simulink model "Roll_Autopilot_PP"  (R2017b)
settings: Solver=FixedStepDiscrete  StartTime=0.0  StopTime=10.0  FixedStep=0.025000  RelTol=1e-3
model workspace (MAT data in the model file):
  MCOS : class17 (value not decoded)
  already_pp = 1
  compositionalMap : struct (value not decoded)
  MCOS : class17 (value not decoded)
  MCOS : class17 (value not decoded)
  verificationResults : struct (value not decoded)
undefined symbols (not defined in the file): contractAfterSimulation, contractBeforeSimulation, ContractBlock, ContractEnsureBlock, ContractGuaranteeBlock, ContractModeBlock, ContractRequireBlock, ContractValidatorBlock, pp_lib, saturation, saveValidatorParameters, slcm, Ts
(part 2 of 3)

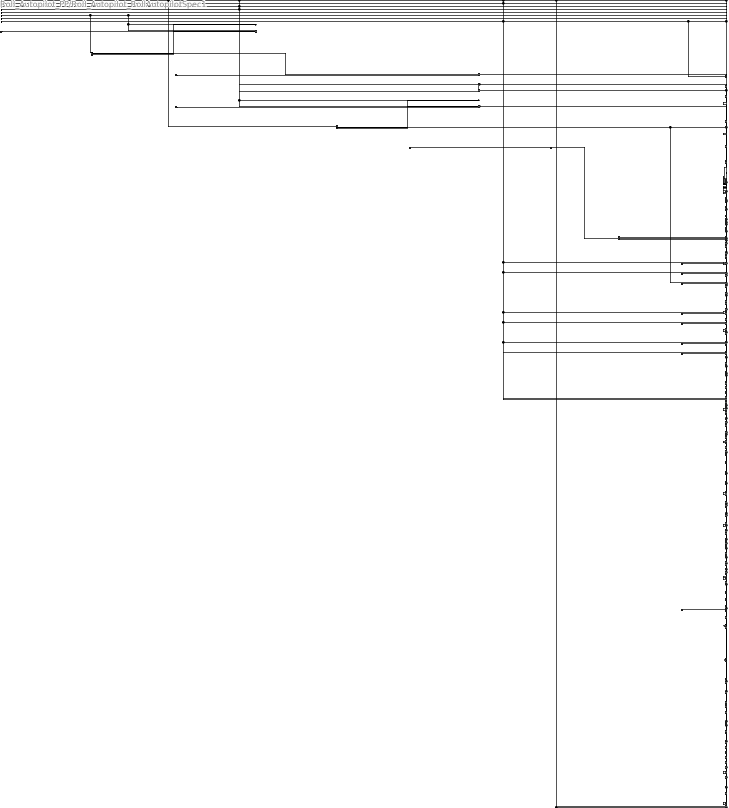
== system Roll_Autopilot_PP/Roll_Autopilot_RollAutopilotSpec1 ==
  note: contract has non-exhaustive modes
  RollAutopilotSpec_roll_angle : Inport  OutDataTypeStr=double
  RollAutopilotSpec_TurnKnob : Inport  Port=2  OutDataTypeStr=double
  RollAutopilotSpec_HDGmode : Inport  Port=3  OutDataTypeStr=boolean
  RollAutopilotSpec_autopilot_engaged : Inport  Port=4  OutDataTypeStr=boolean
  RollAutopilotSpec_hdg_hold_mode_cmd : Inport  Port=5  OutDataTypeStr=double
  RollAutopilotSpec_roll_actuator_command : Inport  Port=6  OutDataTypeStr=double
  RollAutopilotSpec_roll_cmd : Inport  Port=7  OutDataTypeStr=double
  RollAutopilotSpec_roll_hold_reference : Inport  Port=8  OutDataTypeStr=double
  AP_minus_001 : Subsystem  TreatAsAtomicUnit=on  mask(ContractGuaranteeBlock){ContractBlockType=ContractGuaranteeBlock}
      mask init:
      | set_param(gcb, 'LinkStatus', 'none');
      mask DialogControl DescTextVar Prompt: Guarantee block
  AP_minus_003A : Subsystem  TreatAsAtomicUnit=on  mask(ContractGuaranteeBlock){ContractBlockType=ContractGuaranteeBlock}
      mask init:
      | set_param(gcb, 'LinkStatus', 'none');
      mask DialogControl DescTextVar Prompt: Guarantee block
      mask DialogControl Display_counter_example_as_signals Prompt: Display counter example as signals
      mask DialogControl Display_counter_example_as_signals Callback: displayCexSignals(3, 4);displayCexSignals(2,
      mask DialogControl Display_counter_example_as_tables Prompt: Display counter example as tables
      mask DialogControl Display_counter_example_as_tables Callback: displayCexTables(3, 4);displayCexTables(2,
      mask DialogControl Display_counter_example_as_HTML_tables Prompt: Display counter example as HTML tables
      mask DialogControl Display_counter_example_as_HTML_tables Callback: displayCexHtmlTables(3, 4);displayCexHtmlTables(2,
      mask DialogControl Generate_an_outer_model_for_the_counter_example Prompt: Generate an outer model for the counter example
      mask DialogControl Generate_an_outer_model_for_the_counter_example Callback: generateModelWithSignalBuilders(3, 4, 2);generateModelWithSignalBuilders(2,
      mask DialogControl Generate_an_inner_model_for_the_counter_example Prompt: Generate an inner model for the counter example
      mask DialogControl Generate_an_inner_model_for_the_counter_example Callback: generateModelWithSignalBuilders(3, 4, 1);generateModelWithSignalBuilders(2,
  AP_minus_003B : Subsystem  TreatAsAtomicUnit=on  mask(ContractGuaranteeBlock){ContractBlockType=ContractGuaranteeBlock}
      mask init:
      | set_param(gcb, 'LinkStatus', 'none');
      mask DialogControl DescTextVar Prompt: Guarantee block
      mask DialogControl Display_counter_example_as_signals Prompt: Display counter example as signals
      mask DialogControl Display_counter_example_as_signals Callback: displayCexSignals(3, 4);displayCexSignals(1,
      mask DialogControl Display_counter_example_as_tables Prompt: Display counter example as tables
      mask DialogControl Display_counter_example_as_tables Callback: displayCexTables(3, 4);displayCexTables(1,
      mask DialogControl Display_counter_example_as_HTML_tables Prompt: Display counter example as HTML tables
      mask DialogControl Display_counter_example_as_HTML_tables Callback: displayCexHtmlTables(3, 4);displayCexHtmlTables(1,
      mask DialogControl Generate_an_outer_model_for_the_counter_example Prompt: Generate an outer model for the counter example
      mask DialogControl Generate_an_outer_model_for_the_counter_example Callback: generateModelWithSignalBuilders(3, 4, 2);generateModelWithSignalBuilders(1,
      mask DialogControl Generate_an_inner_model_for_the_counter_example Prompt: Generate an inner model for the counter example
      mask DialogControl Generate_an_inner_model_for_the_counter_example Callback: generateModelWithSignalBuilders(3, 4, 1);generateModelWithSignalBuilders(1,
  AP_minus_003C : Subsystem  TreatAsAtomicUnit=on  mask(ContractGuaranteeBlock){ContractBlockType=ContractGuaranteeBlock}
      mask init:
      | set_param(gcb, 'LinkStatus', 'none');
      mask DialogControl DescTextVar Prompt: Guarantee block
      mask DialogControl Display_counter_example_as_signals Prompt: Display counter example as signals
      mask DialogControl Display_counter_example_as_signals Callback: displayCexSignals(3, 4);displayCexSignals(3,
      mask DialogControl Display_counter_example_as_tables Prompt: Display counter example as tables
      mask DialogControl Display_counter_example_as_tables Callback: displayCexTables(3, 4);displayCexTables(3,
      mask DialogControl Display_counter_example_as_HTML_tables Prompt: Display counter example as HTML tables
      mask DialogControl Display_counter_example_as_HTML_tables Callback: displayCexHtmlTables(3, 4);displayCexHtmlTables(3,
      mask DialogControl Generate_an_outer_model_for_the_counter_example Prompt: Generate an outer model for the counter example
      mask DialogControl Generate_an_outer_model_for_the_counter_example Callback: generateModelWithSignalBuilders(3, 4, 2);generateModelWithSignalBuilders(3,
      mask DialogControl Generate_an_inner_model_for_the_counter_example Prompt: Generate an inner model for the counter example
      mask DialogControl Generate_an_inner_model_for_the_counter_example Callback: generateModelWithSignalBuilders(3, 4, 1);generateModelWithSignalBuilders(3,
  AP_minus_003D : Subsystem  TreatAsAtomicUnit=on  mask(ContractGuaranteeBlock){ContractBlockType=ContractGuaranteeBlock}
      mask init:
      | set_param(gcb, 'LinkStatus', 'none');
      mask DialogControl DescTextVar Prompt: Guarantee block
  AP_minus_007 : Subsystem  TreatAsAtomicUnit=on  mask(ContractGuaranteeBlock){ContractBlockType=ContractGuaranteeBlock}
      mask init:
      | set_param(gcb, 'LinkStatus', 'none');
      mask DialogControl DescTextVar Prompt: Guarantee block
  Arrow_xxRollAutopilotSpec_162_ni_7 : Delay  DelayLength=1  InitialCondition=1
  Arrow_xxRollAutopilotSpec_163_ni_9 : Delay  DelayLength=1  InitialCondition=1
  Arrow_xxRollAutopilotSpec_164_ni_12 : Delay  DelayLength=1  InitialCondition=1
  Arrow_xxRollAutopilotSpec_165_ni_16 : Delay  DelayLength=1  InitialCondition=1
  Arrow_xxRollAutopilotSpec_183_ni_3 : Delay  DelayLength=1  InitialCondition=1
  Ca_operator : Logic  Operator=NOT  AllPortsSameDT=off  OutDataTypeStr=boolean
  Cb_operator : Logic  AllPortsSameDT=off  OutDataTypeStr=boolean
  Cc_operator : RelationalOperator  OutDataTypeStr=boolean  RndMeth=Simplest
  Cc_rhs_2 : Constant  Value=30.0  OutDataTypeStr=double
  Cd_operator : Logic  AllPortsSameDT=off  OutDataTypeStr=boolean
  H_call : Subsystem  TreatAsAtomicUnit=on
  H_call1 : Subsystem  TreatAsAtomicUnit=on
  H_call11 : Subsystem  TreatAsAtomicUnit=on
  PRE_xxRollAutopilotSpec_{8,13,17,22,33,38,42,44,59,64,68,73,84,89,93,95,109,114,118,123,133,138,142,144,184,187} (26 alike) : Delay  DelayLength=1  InitialCondition=0
  SI_call : Subsystem  TreatAsAtomicUnit=on
  SI_call1 : Subsystem  TreatAsAtomicUnit=on
  SI_call11 : Subsystem  TreatAsAtomicUnit=on
  SI_call111 : Subsystem  TreatAsAtomicUnit=on
  SI_call1111 : Subsystem  TreatAsAtomicUnit=on
  SI_call11111 : Subsystem  TreatAsAtomicUnit=on
  SI_call111111 : Subsystem  TreatAsAtomicUnit=on
  SI_call1111111 : Subsystem  TreatAsAtomicUnit=on
  SI_call11111111 : Subsystem  TreatAsAtomicUnit=on
  branch_10_IF : Switch  Criteria=u2 ~= 0
  branch_11_IF : Switch  Criteria=u2 ~= 0
  branch_12_IF : Switch  Criteria=u2 ~= 0
  branch_13_IF : Switch  Criteria=u2 ~= 0
  branch_14_IF : Switch  Criteria=u2 ~= 0
  branch_15_IF : Switch  Criteria=u2 ~= 0
  branch_16_IF : Switch  Criteria=u2 ~= 0
  branch_8_IF : Switch  Criteria=u2 ~= 0
  branch_9_IF : Switch  Criteria=u2 ~= 0
  hdg_hold_mode : Subsystem  TreatAsAtomicUnit=on  mask(ContractModeBlock){ContractBlockType=ContractModeBlock}
      mask init:
      | set_param(gcb, 'LinkStatus', 'none');
      mask DialogControl DescTextVar Prompt: Mode block
  hdg_hold_mode_ensure : Subsystem  TreatAsAtomicUnit=on  mask(ContractEnsureBlock){ContractBlockType=ContractEnsureBlock}
      mask init:
      | set_param(gcb, 'LinkStatus', 'none');
      mask DialogControl DescTextVar Prompt: Ensure block
  hdg_hold_mode_ensure_cond : Logic  Inputs=1  AllPortsSameDT=off  OutDataTypeStr=boolean
  hdg_hold_mode_require : Subsystem  TreatAsAtomicUnit=on  mask(ContractRequireBlock){ContractBlockType=ContractRequireBlock}
      mask init:
      | set_param(gcb, 'LinkStatus', 'none');
      mask DialogControl DescTextVar Prompt: Require block
  hdg_hold_mode_require_cond : Logic  Inputs=1  AllPortsSameDT=off  OutDataTypeStr=boolean
  no_other_lateral_mode_operator : Logic  Operator=NOT  AllPortsSameDT=off  OutDataTypeStr=boolean
  roll_hold_mode : Subsystem  TreatAsAtomicUnit=on  mask(ContractModeBlock){ContractBlockType=ContractModeBlock}
      mask init:
      | set_param(gcb, 'LinkStatus', 'none');
      mask DialogControl DescTextVar Prompt: Mode block
  roll_hold_mode_ensure : Subsystem  TreatAsAtomicUnit=on  mask(ContractEnsureBlock){ContractBlockType=ContractEnsureBlock}
      mask init:
      | set_param(gcb, 'LinkStatus', 'none');
      mask DialogControl DescTextVar Prompt: Ensure block
  roll_hold_mode_ensure_cond : Logic  Inputs=1  AllPortsSameDT=off  OutDataTypeStr=boolean
  roll_hold_mode_require : Subsystem  TreatAsAtomicUnit=on  mask(ContractRequireBlock){ContractBlockType=ContractRequireBlock}
      mask init:
      | set_param(gcb, 'LinkStatus', 'none');
      mask DialogControl DescTextVar Prompt: Require block
  roll_hold_mode_require_cond : Logic  Inputs=1  AllPortsSameDT=off  OutDataTypeStr=boolean
  roll_hold_operator : Logic  AllPortsSameDT=off  OutDataTypeStr=boolean
  spec206_operator : Subsystem  TreatAsAtomicUnit=on
  spec211_operator : Logic  AllPortsSameDT=off  OutDataTypeStr=boolean
  spec216_operator : RelationalOperator  Operator===  OutDataTypeStr=boolean  RndMeth=Simplest
  spec223_operator : RelationalOperator  Operator===  OutDataTypeStr=boolean  RndMeth=Simplest
  spec252_operator : Subsystem  TreatAsAtomicUnit=on
  spec621_operator : RelationalOperator  Operator=<=  OutDataTypeStr=boolean  RndMeth=Simplest
  spec621_rhs_2 : Constant  Value=15.0  OutDataTypeStr=double
  validator : M-S-Function  LoadFcn=saveValidatorParameters(gcb);  InitFcn=contractBeforeSimulation();  StopFcn=contractAfterSimulation();  FunctionName=contract  mask(ContractValidatorBlock){assumePorts=0, guaranteePorts=6, modePorts=2, ContractBlockType=ContractValidatorBlock, createInportsCheckbox=off}
      mask prompts: assumePorts "Assume ports     :"; guaranteePorts "Guarantee ports :"; modePorts "Mode ports        :"; createInportsCheckbox "Create inports and connect them automatically"
      mask init:
      | set_param(gcb,'LinkStatus','none');
      | contract_callback('inputs_callback',gcb);
      mask DialogControl DescTextVar Prompt: The validator block implements the following logic: <br> <br> <b>Sofar</b>(assume<sub>1</sub> <b>&#8743;</b> assume<sub>2</sub> <b>&#8743;</b> ... assume<sub>k</sub>) <b>&rarr;</b> (guarantee<sub>1</sub> <b>&#8743;</b> guarantee<sub>2</sub> <b>&#8743;</b> ... guarantee<sub>m</sub> <b>&#8743;</b>  mode<sub>1</sub> <b>&#8743;</b> mode<sub>2</sub> <b>&#8743;</b> ... <b>&#8743;</b> mode<sub>n</sub> )<br> where mode<sub>i</sub> = require<sub>i</sub> <b>&rarr;</b> ensure<sub>i</sub>
      mask DialogControl Display_counter_example_as_signals Prompt: Display counter example as signals
      mask DialogControl Display_counter_example_as_signals Callback: displayCexSignals(2, 1);
      mask DialogControl Display_counter_example_as_tables Prompt: Display counter example as tables
      mask DialogControl Display_counter_example_as_tables Callback: displayCexTables(2, 1);
      mask DialogControl Display_counter_example_as_HTML_tables Prompt: Display counter example as HTML tables
      mask DialogControl Display_counter_example_as_HTML_tables Callback: displayCexHtmlTables(2, 1);
      mask DialogControl Generate_an_outer_model_for_the_counter_example Prompt: Generate an outer model for the counter example
      mask DialogControl Generate_an_outer_model_for_the_counter_example Callback: generateModelWithSignalBuilders(2, 1, 2);
      mask DialogControl Generate_an_inner_model_for_the_counter_example Prompt: Generate an inner model for the counter example
      mask DialogControl Generate_an_inner_model_for_the_counter_example Callback: generateModelWithSignalBuilders(2, 1, 1);
      mask Display:
      | color('black');
      | port_label('input',1,'guarantee');
      | port_label('input',2,'guarantee');
      | port_label('input',3,'guarantee');
      | port_label('input',4,'guarantee');
      | port_label('input',5,'guarantee');
      | port_label('input',6,'guarantee');
      | port_label('input',7,'mode');
      | port_label('input',8,'mode');
      | port_label('output',1,'valid');
  xxRollAutopilotSpec_101_operator : Logic  AllPortsSameDT=off  OutDataTypeStr=boolean
  xxRollAutopilotSpec_102_rhs1 : Constant  Value=true  OutDataTypeStr=boolean
  xxRollAutopilotSpec_104_operator : Product  OutDataTypeStr=double
  xxRollAutopilotSpec_104_rhs_1 : Constant  Value=30.0  OutDataTypeStr=double
  xxRollAutopilotSpec_105_operator : RelationalOperator  Operator===  OutDataTypeStr=boolean  RndMeth=Simplest
  xxRollAutopilotSpec_106_operator : RelationalOperator  OutDataTypeStr=boolean  RndMeth=Simplest
  xxRollAutopilotSpec_106_rhs_2 : Constant  Value=30.0  OutDataTypeStr=double
  xxRollAutopilotSpec_107_operator : Subsystem  TreatAsAtomicUnit=on
  xxRollAutopilotSpec_108_operator : Logic  Operator=NOT  AllPortsSameDT=off  OutDataTypeStr=boolean
  xxRollAutopilotSpec_10_operator : Logic  AllPortsSameDT=off  OutDataTypeStr=boolean
  xxRollAutopilotSpec_110_operator : Logic  Operator=OR  AllPortsSameDT=off  OutDataTypeStr=boolean
  xxRollAutopilotSpec_111_operator : Logic  AllPortsSameDT=off  OutDataTypeStr=boolean
  xxRollAutopilotSpec_112_operator : Subsystem  TreatAsAtomicUnit=on
  xxRollAutopilotSpec_113_operator : Logic  Operator=NOT  AllPortsSameDT=off  OutDataTypeStr=boolean
  xxRollAutopilotSpec_115_operator : Logic  Operator=OR  AllPortsSameDT=off  OutDataTypeStr=boolean
  xxRollAutopilotSpec_116_operator : Logic  AllPortsSameDT=off  OutDataTypeStr=boolean
  xxRollAutopilotSpec_119_operator : Logic  Operator=NOT  AllPortsSameDT=off  OutDataTypeStr=boolean
  xxRollAutopilotSpec_11_operator : Subsystem  TreatAsAtomicUnit=on
  xxRollAutopilotSpec_120_operator : Logic  AllPortsSameDT=off  OutDataTypeStr=boolean
  xxRollAutopilotSpec_121_operator : Logic  Operator=NOT  AllPortsSameDT=off  OutDataTypeStr=boolean
  xxRollAutopilotSpec_122_operator : Logic  Operator=NOT  AllPortsSameDT=off  OutDataTypeStr=boolean
  xxRollAutopilotSpec_124_operator : Logic  Operator=OR  AllPortsSameDT=off  OutDataTypeStr=boolean
  xxRollAutopilotSpec_125_operator : Logic  AllPortsSameDT=off  OutDataTypeStr=boolean
  xxRollAutopilotSpec_127_operator : Subsystem  TreatAsAtomicUnit=on
  xxRollAutopilotSpec_128_operator : Product  OutDataTypeStr=double
  xxRollAutopilotSpec_128_rhs_1 : Constant  Value=30.0  OutDataTypeStr=double
  xxRollAutopilotSpec_129_operator : RelationalOperator  Operator===  OutDataTypeStr=boolean  RndMeth=Simplest
  xxRollAutopilotSpec_12_operator : Logic  Operator=NOT  AllPortsSameDT=off  OutDataTypeStr=boolean
  xxRollAutopilotSpec_130_operator : RelationalOperator  OutDataTypeStr=boolean  RndMeth=Simplest
  xxRollAutopilotSpec_130_rhs_2 : Constant  Value=30.0  OutDataTypeStr=double
  xxRollAutopilotSpec_131_operator : Subsystem  TreatAsAtomicUnit=on
  xxRollAutopilotSpec_132_operator : Logic  Operator=NOT  AllPortsSameDT=off  OutDataTypeStr=boolean
  xxRollAutopilotSpec_134_operator : Logic  Operator=OR  AllPortsSameDT=off  OutDataTypeStr=boolean
  xxRollAutopilotSpec_135_operator : Logic  AllPortsSameDT=off  OutDataTypeStr=boolean
  xxRollAutopilotSpec_136_operator : Subsystem  TreatAsAtomicUnit=on
  xxRollAutopilotSpec_137_operator : Logic  Operator=NOT  AllPortsSameDT=off  OutDataTypeStr=boolean
  xxRollAutopilotSpec_139_operator : Logic  Operator=OR  AllPortsSameDT=off  OutDataTypeStr=boolean
  xxRollAutopilotSpec_140_operator : Logic  AllPortsSameDT=off  OutDataTypeStr=boolean
  xxRollAutopilotSpec_143_operator : Logic  Operator=NOT  AllPortsSameDT=off  OutDataTypeStr=boolean
  xxRollAutopilotSpec_145_operator : Logic  Operator=NOT  AllPortsSameDT=off  OutDataTypeStr=boolean
  xxRollAutopilotSpec_146_operator : Logic  AllPortsSameDT=off  OutDataTypeStr=boolean
  xxRollAutopilotSpec_147_operator : Logic  AllPortsSameDT=off  OutDataTypeStr=boolean
  xxRollAutopilotSpec_148_operator : Subsystem  TreatAsAtomicUnit=on
  xxRollAutopilotSpec_14_operator : Logic  Operator=OR  AllPortsSameDT=off  OutDataTypeStr=boolean
  xxRollAutopilotSpec_150_operator : Logic  AllPortsSameDT=off  OutDataTypeStr=boolean
  xxRollAutopilotSpec_151_rhs1 : Constant  Value=true  OutDataTypeStr=boolean
  xxRollAutopilotSpec_152_operator : RelationalOperator  Operator===  OutDataTypeStr=boolean  RndMeth=Simplest
  xxRollAutopilotSpec_153_operator : RelationalOperator  OutDataTypeStr=boolean  RndMeth=Simplest
  xxRollAutopilotSpec_153_rhs_2 : Constant  Value=-30.0  OutDataTypeStr=double
  xxRollAutopilotSpec_154_operator : RelationalOperator  Operator=<=  OutDataTypeStr=boolean  RndMeth=Simplest
  xxRollAutopilotSpec_154_rhs_2 : Constant  Value=30.0  OutDataTypeStr=double
  xxRollAutopilotSpec_155_operator : Logic  Operator=OR  AllPortsSameDT=off  OutDataTypeStr=boolean
  xxRollAutopilotSpec_156_operator : RelationalOperator  Operator=<=  OutDataTypeStr=boolean  RndMeth=Simplest
  xxRollAutopilotSpec_156_rhs_2 : Constant  Value=-3.0  OutDataTypeStr=double
  xxRollAutopilotSpec_157_operator : RelationalOperator  OutDataTypeStr=boolean  RndMeth=Simplest
  xxRollAutopilotSpec_157_rhs_2 : Constant  Value=3.0  OutDataTypeStr=double
  xxRollAutopilotSpec_158_operator : Logic  Operator=OR  AllPortsSameDT=off  OutDataTypeStr=boolean
  xxRollAutopilotSpec_159_operator : Logic  AllPortsSameDT=off  OutDataTypeStr=boolean
  xxRollAutopilotSpec_15_operator : Logic  AllPortsSameDT=off  OutDataTypeStr=boolean
  xxRollAutopilotSpec_160_operator : RelationalOperator  Operator===  OutDataTypeStr=boolean  RndMeth=Simplest
  xxRollAutopilotSpec_160_rhs_2 : Constant  Value=0.0  OutDataTypeStr=double
  xxRollAutopilotSpec_161_operator : Logic  Operator=NOT  AllPortsSameDT=off  OutDataTypeStr=boolean
  xxRollAutopilotSpec_162_ni_7_init : Constant  Value=0  OutDataTypeStr=boolean
  xxRollAutopilotSpec_163_ni_9_init : Constant  Value=0  OutDataTypeStr=boolean
  xxRollAutopilotSpec_164_ni_12_init : Constant  Value=0  OutDataTypeStr=boolean
  xxRollAutopilotSpec_165_ni_16_init : Constant  Value=0  OutDataTypeStr=boolean
  xxRollAutopilotSpec_166_rhs : Constant  Value=false  OutDataTypeStr=boolean
  xxRollAutopilotSpec_166_rhs1 : Constant  Value=true  OutDataTypeStr=boolean
  xxRollAutopilotSpec_167_operator : RelationalOperator  OutDataTypeStr=boolean  RndMeth=Simplest
  xxRollAutopilotSpec_167_rhs_2 : Constant  Value=0.0  OutDataTypeStr=double
  xxRollAutopilotSpec_168_operator : Gain  Gain=-1  OutDataTypeStr=double
  xxRollAutopilotSpec_169_operator : RelationalOperator  OutDataTypeStr=boolean  RndMeth=Simplest
  xxRollAutopilotSpec_169_rhs_2 : Constant  Value=0.0  OutDataTypeStr=double
  xxRollAutopilotSpec_170_operator : Gain  Gain=-1  OutDataTypeStr=double
  xxRollAutopilotSpec_171_rhs : Constant  Value=1.0  OutDataTypeStr=double
  xxRollAutopilotSpec_172_rhs : Constant  Value=-1.0  OutDataTypeStr=double
  xxRollAutopilotSpec_173_operator : RelationalOperator  Operator=<  OutDataTypeStr=boolean  RndMeth=Simplest
  xxRollAutopilotSpec_173_rhs_2 : Constant  Value=6.0  OutDataTypeStr=double
  xxRollAutopilotSpec_174_operator : RelationalOperator  Operator=>  OutDataTypeStr=boolean  RndMeth=Simplest
  xxRollAutopilotSpec_174_rhs_2 : Constant  Value=-6.0  OutDataTypeStr=double
  xxRollAutopilotSpec_175_operator : RelationalOperator  OutDataTypeStr=boolean  RndMeth=Simplest
  xxRollAutopilotSpec_175_rhs_2 : Constant  Value=-30.0  OutDataTypeStr=double
  xxRollAutopilotSpec_176_operator : RelationalOperator  Operator=<=  OutDataTypeStr=boolean  RndMeth=Simplest
  xxRollAutopilotSpec_176_rhs_2 : Constant  Value=30.0  OutDataTypeStr=double
  xxRollAutopilotSpec_177_operator : Logic  Operator=OR  AllPortsSameDT=off  OutDataTypeStr=boolean
  xxRollAutopilotSpec_178_operator : RelationalOperator  Operator=<=  OutDataTypeStr=boolean  RndMeth=Simplest
  xxRollAutopilotSpec_178_rhs_2 : Constant  Value=-3.0  OutDataTypeStr=double
  xxRollAutopilotSpec_179_operator : RelationalOperator  OutDataTypeStr=boolean  RndMeth=Simplest
  xxRollAutopilotSpec_179_rhs_2 : Constant  Value=3.0  OutDataTypeStr=double
  xxRollAutopilotSpec_180_operator : Logic  Operator=OR  AllPortsSameDT=off  OutDataTypeStr=boolean
  xxRollAutopilotSpec_181_operator : Logic  Operator=OR  AllPortsSameDT=off  OutDataTypeStr=boolean
  xxRollAutopilotSpec_182_operator : Logic  Operator=OR  AllPortsSameDT=off  OutDataTypeStr=boolean
  xxRollAutopilotSpec_183_ni_3_init : Constant  Value=0  OutDataTypeStr=boolean
  xxRollAutopilotSpec_185_rhs1 : Constant  Value=false  OutDataTypeStr=boolean
  xxRollAutopilotSpec_186_rhs : Constant  Value=0.0  OutDataTypeStr=double
  xxRollAutopilotSpec_18_operator : Logic  Operator=NOT  AllPortsSameDT=off  OutDataTypeStr=boolean
  xxRollAutopilotSpec_19_operator : Logic  AllPortsSameDT=off  OutDataTypeStr=boolean
  xxRollAutopilotSpec_20_operator : Logic  Operator=NOT  AllPortsSameDT=off  OutDataTypeStr=boolean
  xxRollAutopilotSpec_21_operator : Logic  Operator=NOT  AllPortsSameDT=off  OutDataTypeStr=boolean
  xxRollAutopilotSpec_23_operator : Logic  Operator=OR  AllPortsSameDT=off  OutDataTypeStr=boolean
  xxRollAutopilotSpec_24_operator : Logic  AllPortsSameDT=off  OutDataTypeStr=boolean
  xxRollAutopilotSpec_26_operator : Subsystem  TreatAsAtomicUnit=on
  xxRollAutopilotSpec_27_operator : RelationalOperator  Operator===  OutDataTypeStr=boolean  RndMeth=Simplest
  xxRollAutopilotSpec_28_operator : Logic  Operator=OR  AllPortsSameDT=off  OutDataTypeStr=boolean
  xxRollAutopilotSpec_29_operator : Logic  Operator=OR  AllPortsSameDT=off  OutDataTypeStr=boolean
  xxRollAutopilotSpec_2_operator : RelationalOperator  Operator===  OutDataTypeStr=boolean  RndMeth=Simplest
  xxRollAutopilotSpec_30_operator : Logic  Operator=NOT  AllPortsSameDT=off  OutDataTypeStr=boolean
  xxRollAutopilotSpec_31_operator : Subsystem  TreatAsAtomicUnit=on
  xxRollAutopilotSpec_32_operator : Logic  Operator=NOT  AllPortsSameDT=off  OutDataTypeStr=boolean
  xxRollAutopilotSpec_34_operator : Logic  Operator=OR  AllPortsSameDT=off  OutDataTypeStr=boolean
  xxRollAutopilotSpec_35_operator : Logic  AllPortsSameDT=off  OutDataTypeStr=boolean
  xxRollAutopilotSpec_36_operator : Subsystem  TreatAsAtomicUnit=on
  xxRollAutopilotSpec_37_operator : Logic  Operator=NOT  AllPortsSameDT=off  OutDataTypeStr=boolean
  xxRollAutopilotSpec_39_operator : Logic  Operator=OR  AllPortsSameDT=off  OutDataTypeStr=boolean
  xxRollAutopilotSpec_3_operator : Logic  Operator=OR  AllPortsSameDT=off  OutDataTypeStr=boolean
  xxRollAutopilotSpec_40_operator : Logic  AllPortsSameDT=off  OutDataTypeStr=boolean
  xxRollAutopilotSpec_43_operator : Logic  Operator=NOT  AllPortsSameDT=off  OutDataTypeStr=boolean
  xxRollAutopilotSpec_45_operator : Logic  Operator=NOT  AllPortsSameDT=off  OutDataTypeStr=boolean
  xxRollAutopilotSpec_46_operator : Logic  AllPortsSameDT=off  OutDataTypeStr=boolean
  xxRollAutopilotSpec_47_operator : Logic  AllPortsSameDT=off  OutDataTypeStr=boolean
  xxRollAutopilotSpec_48_operator : Subsystem  TreatAsAtomicUnit=on
  xxRollAutopilotSpec_4_operator : Logic  Operator=OR  AllPortsSameDT=off  OutDataTypeStr=boolean
  xxRollAutopilotSpec_50_operator : Logic  AllPortsSameDT=off  OutDataTypeStr=boolean
  xxRollAutopilotSpec_51_rhs1 : Constant  Value=true  OutDataTypeStr=boolean
  xxRollAutopilotSpec_53_operator : RelationalOperator  Operator===  OutDataTypeStr=boolean  RndMeth=Simplest
  xxRollAutopilotSpec_53_rhs_2 : Constant  Value=0.0  OutDataTypeStr=double
  xxRollAutopilotSpec_54_operator : RelationalOperator  Operator=>  OutDataTypeStr=boolean  RndMeth=Simplest
  xxRollAutopilotSpec_54_rhs_2 : Constant  Value=-6.0  OutDataTypeStr=double
  xxRollAutopilotSpec_55_operator : RelationalOperator  Operator=<  OutDataTypeStr=boolean  RndMeth=Simplest
  xxRollAutopilotSpec_55_rhs_2 : Constant  Value=6.0  OutDataTypeStr=double
  xxRollAutopilotSpec_56_operator : Logic  AllPortsSameDT=off  OutDataTypeStr=boolean
  xxRollAutopilotSpec_57_operator : Subsystem  TreatAsAtomicUnit=on
  xxRollAutopilotSpec_58_operator : Logic  Operator=NOT  AllPortsSameDT=off  OutDataTypeStr=boolean
  xxRollAutopilotSpec_5_operator : Logic  Operator=NOT  AllPortsSameDT=off  OutDataTypeStr=boolean
  xxRollAutopilotSpec_60_operator : Logic  Operator=OR  AllPortsSameDT=off  OutDataTypeStr=boolean
  xxRollAutopilotSpec_61_operator : Logic  AllPortsSameDT=off  OutDataTypeStr=boolean
  xxRollAutopilotSpec_62_operator : Subsystem  TreatAsAtomicUnit=on
  xxRollAutopilotSpec_63_operator : Logic  Operator=NOT  AllPortsSameDT=off  OutDataTypeStr=boolean
  xxRollAutopilotSpec_65_operator : Logic  Operator=OR  AllPortsSameDT=off  OutDataTypeStr=boolean
  xxRollAutopilotSpec_66_operator : Logic  AllPortsSameDT=off  OutDataTypeStr=boolean
  xxRollAutopilotSpec_69_operator : Logic  Operator=NOT  AllPortsSameDT=off  OutDataTypeStr=boolean
  xxRollAutopilotSpec_6_operator : Subsystem  TreatAsAtomicUnit=on
  xxRollAutopilotSpec_70_operator : Logic  AllPortsSameDT=off  OutDataTypeStr=boolean
  xxRollAutopilotSpec_71_operator : Logic  Operator=NOT  AllPortsSameDT=off  OutDataTypeStr=boolean
  xxRollAutopilotSpec_72_operator : Logic  Operator=NOT  AllPortsSameDT=off  OutDataTypeStr=boolean
  xxRollAutopilotSpec_74_operator : Logic  Operator=OR  AllPortsSameDT=off  OutDataTypeStr=boolean
  xxRollAutopilotSpec_75_operator : Logic  AllPortsSameDT=off  OutDataTypeStr=boolean
  xxRollAutopilotSpec_77_operator : Subsystem  TreatAsAtomicUnit=on
  xxRollAutopilotSpec_78_operator : RelationalOperator  Operator===  OutDataTypeStr=boolean  RndMeth=Simplest
  xxRollAutopilotSpec_78_rhs_2 : Constant  Value=0.0  OutDataTypeStr=double
  xxRollAutopilotSpec_79_operator : RelationalOperator  Operator=>  OutDataTypeStr=boolean  RndMeth=Simplest
  xxRollAutopilotSpec_79_rhs_2 : Constant  Value=-6.0  OutDataTypeStr=double
  xxRollAutopilotSpec_7_operator : Logic  Operator=NOT  AllPortsSameDT=off  OutDataTypeStr=boolean
  xxRollAutopilotSpec_80_operator : RelationalOperator  Operator=<  OutDataTypeStr=boolean  RndMeth=Simplest
  xxRollAutopilotSpec_80_rhs_2 : Constant  Value=6.0  OutDataTypeStr=double
  xxRollAutopilotSpec_81_operator : Logic  AllPortsSameDT=off  OutDataTypeStr=boolean
  xxRollAutopilotSpec_82_operator : Subsystem  TreatAsAtomicUnit=on
  xxRollAutopilotSpec_83_operator : Logic  Operator=NOT  AllPortsSameDT=off  OutDataTypeStr=boolean
  xxRollAutopilotSpec_85_operator : Logic  Operator=OR  AllPortsSameDT=off  OutDataTypeStr=boolean
  xxRollAutopilotSpec_86_operator : Logic  AllPortsSameDT=off  OutDataTypeStr=boolean
  xxRollAutopilotSpec_87_operator : Subsystem  TreatAsAtomicUnit=on
  xxRollAutopilotSpec_88_operator : Logic  Operator=NOT  AllPortsSameDT=off  OutDataTypeStr=boolean
  xxRollAutopilotSpec_90_operator : Logic  Operator=OR  AllPortsSameDT=off  OutDataTypeStr=boolean
  xxRollAutopilotSpec_91_operator : Logic  AllPortsSameDT=off  OutDataTypeStr=boolean
  xxRollAutopilotSpec_94_operator : Logic  Operator=NOT  AllPortsSameDT=off  OutDataTypeStr=boolean
  xxRollAutopilotSpec_96_operator : Logic  Operator=NOT  AllPortsSameDT=off  OutDataTypeStr=boolean
  xxRollAutopilotSpec_97_operator : Logic  AllPortsSameDT=off  OutDataTypeStr=boolean
  xxRollAutopilotSpec_98_operator : Logic  AllPortsSameDT=off  OutDataTypeStr=boolean
  xxRollAutopilotSpec_99_operator : Subsystem  TreatAsAtomicUnit=on
  xxRollAutopilotSpec_9_operator : Logic  Operator=OR  AllPortsSameDT=off  OutDataTypeStr=boolean
  valid : Outport
  wires:
  validator/1 -> valid/1
  PRE_xxRollAutopilotSpec_8/1 -> xxRollAutopilotSpec_9_operator/2
  PRE_xxRollAutopilotSpec_93/1 -> xxRollAutopilotSpec_99_operator/2(B)
  xxRollAutopilotSpec_98_operator/1 -> xxRollAutopilotSpec_99_operator/1(A)
  xxRollAutopilotSpec_94_operator/1 -> xxRollAutopilotSpec_98_operator/2
  xxRollAutopilotSpec_97_operator/1 -> xxRollAutopilotSpec_98_operator/1
  PRE_xxRollAutopilotSpec_95/1 -> xxRollAutopilotSpec_97_operator/2
  xxRollAutopilotSpec_96_operator/1 -> xxRollAutopilotSpec_97_operator/1
  xxRollAutopilotSpec_90_operator/1 -> xxRollAutopilotSpec_91_operator/2
  PRE_xxRollAutopilotSpec_89/1 -> xxRollAutopilotSpec_90_operator/2
  xxRollAutopilotSpec_82_operator/1(A_equal__equal__gt_B) -> xxRollAutopilotSpec_87_operator/2(B)
  xxRollAutopilotSpec_86_operator/1 -> xxRollAutopilotSpec_87_operator/1(A)
  xxRollAutopilotSpec_85_operator/1 -> xxRollAutopilotSpec_86_operator/2
  PRE_xxRollAutopilotSpec_84/1 -> xxRollAutopilotSpec_85_operator/2
  xxRollAutopilotSpec_78_operator/1 -> xxRollAutopilotSpec_82_operator/2(B)
  xxRollAutopilotSpec_81_operator/1 -> xxRollAutopilotSpec_82_operator/1(A)
  xxRollAutopilotSpec_79_operator/1 -> xxRollAutopilotSpec_81_operator/2
  xxRollAutopilotSpec_80_operator/1 -> xxRollAutopilotSpec_81_operator/1
  xxRollAutopilotSpec_80_rhs_2/1 -> xxRollAutopilotSpec_80_operator/2
  xxRollAutopilotSpec_79_rhs_2/1 -> xxRollAutopilotSpec_79_operator/2
  xxRollAutopilotSpec_78_rhs_2/1 -> xxRollAutopilotSpec_78_operator/2
  SI_call111/1(SI_Z) -> xxRollAutopilotSpec_77_operator/2(B)
  SI_call11/1(SI_Z) -> xxRollAutopilotSpec_77_operator/1(A)
  xxRollAutopilotSpec_74_operator/1 -> xxRollAutopilotSpec_75_operator/2
  PRE_xxRollAutopilotSpec_73/1 -> xxRollAutopilotSpec_74_operator/2
  xxRollAutopilotSpec_70_operator/1 -> xxRollAutopilotSpec_71_operator/1
  PRE_xxRollAutopilotSpec_68/1 -> xxRollAutopilotSpec_70_operator/2
  xxRollAutopilotSpec_69_operator/1 -> xxRollAutopilotSpec_70_operator/1
  xxRollAutopilotSpec_2_operator/1 -> xxRollAutopilotSpec_6_operator/2(B)
  xxRollAutopilotSpec_5_operator/1 -> xxRollAutopilotSpec_6_operator/1(A)
  xxRollAutopilotSpec_65_operator/1 -> xxRollAutopilotSpec_66_operator/2
  PRE_xxRollAutopilotSpec_64/1 -> xxRollAutopilotSpec_65_operator/2
  xxRollAutopilotSpec_57_operator/1(A_equal__equal__gt_B) -> xxRollAutopilotSpec_62_operator/2(B)
  xxRollAutopilotSpec_61_operator/1 -> xxRollAutopilotSpec_62_operator/1(A)
  xxRollAutopilotSpec_60_operator/1 -> xxRollAutopilotSpec_61_operator/2
  PRE_xxRollAutopilotSpec_59/1 -> xxRollAutopilotSpec_60_operator/2
  xxRollAutopilotSpec_4_operator/1 -> xxRollAutopilotSpec_5_operator/1
  xxRollAutopilotSpec_53_operator/1 -> xxRollAutopilotSpec_57_operator/2(B)
  xxRollAutopilotSpec_56_operator/1 -> xxRollAutopilotSpec_57_operator/1(A)
  xxRollAutopilotSpec_54_operator/1 -> xxRollAutopilotSpec_56_operator/2
  xxRollAutopilotSpec_55_operator/1 -> xxRollAutopilotSpec_56_operator/1
  xxRollAutopilotSpec_55_rhs_2/1 -> xxRollAutopilotSpec_55_operator/2
  xxRollAutopilotSpec_54_rhs_2/1 -> xxRollAutopilotSpec_54_operator/2
  xxRollAutopilotSpec_53_rhs_2/1 -> xxRollAutopilotSpec_53_operator/2
  xxRollAutopilotSpec_26_operator/1(A_equal__equal__gt_B) -> xxRollAutopilotSpec_50_operator/2
  H_call/1(H_Y) -> xxRollAutopilotSpec_50_operator/1
  xxRollAutopilotSpec_3_operator/1 -> xxRollAutopilotSpec_4_operator/1
  PRE_xxRollAutopilotSpec_42/1 -> xxRollAutopilotSpec_48_operator/2(B)
  xxRollAutopilotSpec_47_operator/1 -> xxRollAutopilotSpec_48_operator/1(A)
  xxRollAutopilotSpec_43_operator/1 -> xxRollAutopilotSpec_47_operator/2
  xxRollAutopilotSpec_46_operator/1 -> xxRollAutopilotSpec_47_operator/1
  PRE_xxRollAutopilotSpec_44/1 -> xxRollAutopilotSpec_46_operator/2
  xxRollAutopilotSpec_45_operator/1 -> xxRollAutopilotSpec_46_operator/1
  xxRollAutopilotSpec_39_operator/1 -> xxRollAutopilotSpec_40_operator/2
  PRE_xxRollAutopilotSpec_38/1 -> xxRollAutopilotSpec_39_operator/2
  xxRollAutopilotSpec_31_operator/1(A_equal__equal__gt_B) -> xxRollAutopilotSpec_36_operator/2(B)
  xxRollAutopilotSpec_35_operator/1 -> xxRollAutopilotSpec_36_operator/1(A)
  xxRollAutopilotSpec_34_operator/1 -> xxRollAutopilotSpec_35_operator/2
  PRE_xxRollAutopilotSpec_33/1 -> xxRollAutopilotSpec_34_operator/2
  xxRollAutopilotSpec_27_operator/1 -> xxRollAutopilotSpec_31_operator/2(B)
  xxRollAutopilotSpec_30_operator/1 -> xxRollAutopilotSpec_31_operator/1(A)
  xxRollAutopilotSpec_29_operator/1 -> xxRollAutopilotSpec_30_operator/1
  xxRollAutopilotSpec_28_operator/1 -> xxRollAutopilotSpec_29_operator/1
  SI_call1/1(SI_Z) -> xxRollAutopilotSpec_26_operator/2(B)
  SI_call/1(SI_Z) -> xxRollAutopilotSpec_26_operator/1(A)
  xxRollAutopilotSpec_23_operator/1 -> xxRollAutopilotSpec_24_operator/2
  PRE_xxRollAutopilotSpec_22/1 -> xxRollAutopilotSpec_23_operator/2
  xxRollAutopilotSpec_19_operator/1 -> xxRollAutopilotSpec_20_operator/1
  PRE_xxRollAutopilotSpec_17/1 -> xxRollAutopilotSpec_19_operator/2
  xxRollAutopilotSpec_18_operator/1 -> xxRollAutopilotSpec_19_operator/1
  xxRollAutopilotSpec_181_operator/1 -> xxRollAutopilotSpec_182_operator/1
  xxRollAutopilotSpec_178_operator/1 -> xxRollAutopilotSpec_180_operator/2
  xxRollAutopilotSpec_179_operator/1 -> xxRollAutopilotSpec_180_operator/1
  xxRollAutopilotSpec_179_rhs_2/1 -> xxRollAutopilotSpec_179_operator/2
  xxRollAutopilotSpec_178_rhs_2/1 -> xxRollAutopilotSpec_178_operator/2
  xxRollAutopilotSpec_175_operator/1 -> xxRollAutopilotSpec_177_operator/2
  xxRollAutopilotSpec_176_operator/1 -> xxRollAutopilotSpec_177_operator/1
  xxRollAutopilotSpec_176_rhs_2/1 -> xxRollAutopilotSpec_176_operator/2
  xxRollAutopilotSpec_175_rhs_2/1 -> xxRollAutopilotSpec_175_operator/2
  xxRollAutopilotSpec_174_rhs_2/1 -> xxRollAutopilotSpec_174_operator/2
  xxRollAutopilotSpec_173_rhs_2/1 -> xxRollAutopilotSpec_173_operator/2
  xxRollAutopilotSpec_169_rhs_2/1 -> xxRollAutopilotSpec_169_operator/2
  xxRollAutopilotSpec_167_rhs_2/1 -> xxRollAutopilotSpec_167_operator/2
  xxRollAutopilotSpec_160_rhs_2/1 -> xxRollAutopilotSpec_160_operator/2
  xxRollAutopilotSpec_14_operator/1 -> xxRollAutopilotSpec_15_operator/2
  xxRollAutopilotSpec_155_operator/1 -> xxRollAutopilotSpec_159_operator/2
  xxRollAutopilotSpec_158_operator/1 -> xxRollAutopilotSpec_159_operator/1
  xxRollAutopilotSpec_156_operator/1 -> xxRollAutopilotSpec_158_operator/2
  xxRollAutopilotSpec_157_operator/1 -> xxRollAutopilotSpec_158_operator/1
  xxRollAutopilotSpec_157_rhs_2/1 -> xxRollAutopilotSpec_157_operator/2
  xxRollAutopilotSpec_156_rhs_2/1 -> xxRollAutopilotSpec_156_operator/2
  xxRollAutopilotSpec_153_operator/1 -> xxRollAutopilotSpec_155_operator/2
  xxRollAutopilotSpec_154_operator/1 -> xxRollAutopilotSpec_155_operator/1
  xxRollAutopilotSpec_154_rhs_2/1 -> xxRollAutopilotSpec_154_operator/2
  xxRollAutopilotSpec_153_rhs_2/1 -> xxRollAutopilotSpec_153_operator/2
  xxRollAutopilotSpec_127_operator/1(A_equal__equal__gt_B) -> xxRollAutopilotSpec_150_operator/2
  H_call11/1(H_Y) -> xxRollAutopilotSpec_150_operator/1
  PRE_xxRollAutopilotSpec_13/1 -> xxRollAutopilotSpec_14_operator/2
  PRE_xxRollAutopilotSpec_142/1 -> xxRollAutopilotSpec_148_operator/2(B)
  xxRollAutopilotSpec_147_operator/1 -> xxRollAutopilotSpec_148_operator/1(A)
  xxRollAutopilotSpec_143_operator/1 -> xxRollAutopilotSpec_147_operator/2
  xxRollAutopilotSpec_146_operator/1 -> xxRollAutopilotSpec_147_operator/1
  PRE_xxRollAutopilotSpec_144/1 -> xxRollAutopilotSpec_146_operator/2
  xxRollAutopilotSpec_145_operator/1 -> xxRollAutopilotSpec_146_operator/1
  xxRollAutopilotSpec_139_operator/1 -> xxRollAutopilotSpec_140_operator/2
  PRE_xxRollAutopilotSpec_138/1 -> xxRollAutopilotSpec_139_operator/2
  xxRollAutopilotSpec_131_operator/1(A_equal__equal__gt_B) -> xxRollAutopilotSpec_136_operator/2(B)
  xxRollAutopilotSpec_135_operator/1 -> xxRollAutopilotSpec_136_operator/1(A)
  xxRollAutopilotSpec_134_operator/1 -> xxRollAutopilotSpec_135_operator/2
  PRE_xxRollAutopilotSpec_133/1 -> xxRollAutopilotSpec_134_operator/2
  xxRollAutopilotSpec_129_operator/1 -> xxRollAutopilotSpec_131_operator/2(B)
  xxRollAutopilotSpec_130_operator/1 -> xxRollAutopilotSpec_131_operator/1(A)
  xxRollAutopilotSpec_130_rhs_2/1 -> xxRollAutopilotSpec_130_operator/2
  xxRollAutopilotSpec_128_operator/1 -> xxRollAutopilotSpec_129_operator/2
  xxRollAutopilotSpec_128_rhs_1/1 -> xxRollAutopilotSpec_128_operator/1
  SI_call11111/1(SI_Z) -> xxRollAutopilotSpec_127_operator/2(B)
  SI_call1111/1(SI_Z) -> xxRollAutopilotSpec_127_operator/1(A)
  xxRollAutopilotSpec_124_operator/1 -> xxRollAutopilotSpec_125_operator/2
  PRE_xxRollAutopilotSpec_123/1 -> xxRollAutopilotSpec_124_operator/2
  xxRollAutopilotSpec_120_operator/1 -> xxRollAutopilotSpec_121_operator/1
  PRE_xxRollAutopilotSpec_118/1 -> xxRollAutopilotSpec_120_operator/2
  xxRollAutopilotSpec_119_operator/1 -> xxRollAutopilotSpec_120_operator/1
  xxRollAutopilotSpec_6_operator/1(A_equal__equal__gt_B) -> xxRollAutopilotSpec_11_operator/2(B)
  xxRollAutopilotSpec_10_operator/1 -> xxRollAutopilotSpec_11_operator/1(A)
  xxRollAutopilotSpec_115_operator/1 -> xxRollAutopilotSpec_116_operator/2
  PRE_xxRollAutopilotSpec_114/1 -> xxRollAutopilotSpec_115_operator/2
  xxRollAutopilotSpec_107_operator/1(A_equal__equal__gt_B) -> xxRollAutopilotSpec_112_operator/2(B)
  xxRollAutopilotSpec_111_operator/1 -> xxRollAutopilotSpec_112_operator/1(A)
  xxRollAutopilotSpec_110_operator/1 -> xxRollAutopilotSpec_111_operator/2
  PRE_xxRollAutopilotSpec_109/1 -> xxRollAutopilotSpec_110_operator/2
  xxRollAutopilotSpec_9_operator/1 -> xxRollAutopilotSpec_10_operator/2
  xxRollAutopilotSpec_105_operator/1 -> xxRollAutopilotSpec_107_operator/2(B)
  xxRollAutopilotSpec_106_operator/1 -> xxRollAutopilotSpec_107_operator/1(A)
  xxRollAutopilotSpec_106_rhs_2/1 -> xxRollAutopilotSpec_106_operator/2
  xxRollAutopilotSpec_104_operator/1 -> xxRollAutopilotSpec_105_operator/2
  xxRollAutopilotSpec_104_rhs_1/1 -> xxRollAutopilotSpec_104_operator/1
  xxRollAutopilotSpec_77_operator/1(A_equal__equal__gt_B) -> xxRollAutopilotSpec_101_operator/2
  H_call1/1(H_Y) -> xxRollAutopilotSpec_101_operator/1
  hdg_hold_mode/1(mode) -> validator/8
  roll_hold_mode/1(mode) -> validator/7
  AP_minus_007/1(guarantee) -> validator/6
  AP_minus_003A/1(guarantee) -> validator/5
  AP_minus_003B/1(guarantee) -> validator/4
  AP_minus_003C/1(guarantee) -> validator/3
  AP_minus_003D/1(guarantee) -> validator/2
  AP_minus_001/1(guarantee) -> validator/1
  spec621_rhs_2/1 -> spec621_operator/2
  branch_8_IF/1 -> spec621_operator/1
  xxRollAutopilotSpec_152_operator/1 -> spec252_operator/2(B)
  xxRollAutopilotSpec_159_operator/1 -> spec252_operator/1(A)
  RollAutopilotSpec_hdg_hold_mode_cmd/1 -> spec223_operator/2
  xxRollAutopilotSpec_160_operator/1 -> spec206_operator/2(B)
  xxRollAutopilotSpec_161_operator/1 -> spec206_operator/1(A)
  spec211_operator/1 -> roll_hold_mode_require_cond/1
  roll_hold_mode_require_cond/1 -> roll_hold_mode_require/1(In1)
  spec216_operator/1 -> roll_hold_mode_ensure_cond/1
  roll_hold_mode_ensure_cond/1 -> roll_hold_mode_ensure/1(In1)
  roll_hold_mode_ensure/1(ensure) -> roll_hold_mode/2(ensure)
  roll_hold_mode_require/1(require) -> roll_hold_mode/1(require)
  branch_15_IF/1 -> [RollAutopilotSpec_pre_roll_angle]
  branch_16_IF/1 -> [RollAutopilotSpec_pre_Ca]
  hdg_hold_mode_require_cond/1 -> hdg_hold_mode_require/1(In1)
  spec223_operator/1 -> hdg_hold_mode_ensure_cond/1
  hdg_hold_mode_ensure_cond/1 -> hdg_hold_mode_ensure/1(In1)
  hdg_hold_mode_ensure/1(ensure) -> hdg_hold_mode/2(ensure)
  hdg_hold_mode_require/1(require) -> hdg_hold_mode/1(require)
  xxRollAutopilotSpec_170_operator/1 -> branch_9_IF/3
  xxRollAutopilotSpec_168_operator/1 -> branch_8_IF/3
  xxRollAutopilotSpec_167_operator/1 -> branch_8_IF/2
  PRE_xxRollAutopilotSpec_184/1 -> branch_16_IF/3
  xxRollAutopilotSpec_185_rhs1/1 -> branch_16_IF/1
  PRE_xxRollAutopilotSpec_187/1 -> branch_15_IF/3
  xxRollAutopilotSpec_186_rhs/1 -> branch_15_IF/1
  xxRollAutopilotSpec_150_operator/1 -> branch_14_IF/3
  Arrow_xxRollAutopilotSpec_162_ni_7/1 -> branch_14_IF/2
  xxRollAutopilotSpec_151_rhs1/1 -> branch_14_IF/1
  xxRollAutopilotSpec_172_rhs/1 -> branch_13_IF/3
  xxRollAutopilotSpec_171_rhs/1 -> branch_13_IF/1
  xxRollAutopilotSpec_101_operator/1 -> branch_12_IF/3
  Arrow_xxRollAutopilotSpec_163_ni_9/1 -> branch_12_IF/2
  xxRollAutopilotSpec_102_rhs1/1 -> branch_12_IF/1
  xxRollAutopilotSpec_50_operator/1 -> branch_11_IF/3
  Arrow_xxRollAutopilotSpec_164_ni_12/1 -> branch_11_IF/2
  xxRollAutopilotSpec_51_rhs1/1 -> branch_11_IF/1
  xxRollAutopilotSpec_166_rhs/1 -> branch_10_IF/3
  Arrow_xxRollAutopilotSpec_165_ni_16/1 -> branch_10_IF/2
  xxRollAutopilotSpec_166_rhs1/1 -> branch_10_IF/1
  xxRollAutopilotSpec_136_operator/1(A_equal__equal__gt_B) -> SI_call11111111/2(SI_Y)
  xxRollAutopilotSpec_140_operator/1 -> SI_call11111111/1(SI_X)
  xxRollAutopilotSpec_36_operator/1(A_equal__equal__gt_B) -> SI_call1111111/2(SI_Y)
  xxRollAutopilotSpec_40_operator/1 -> SI_call1111111/1(SI_X)
  xxRollAutopilotSpec_87_operator/1(A_equal__equal__gt_B) -> SI_call111111/2(SI_Y)
  xxRollAutopilotSpec_91_operator/1 -> SI_call111111/1(SI_X)
  xxRollAutopilotSpec_112_operator/1(A_equal__equal__gt_B) -> SI_call11111/2(SI_Y)
  xxRollAutopilotSpec_116_operator/1 -> SI_call11111/1(SI_X)
  xxRollAutopilotSpec_121_operator/1 -> SI_call1111/2(SI_Y)
  xxRollAutopilotSpec_125_operator/1 -> SI_call1111/1(SI_X)
  xxRollAutopilotSpec_62_operator/1(A_equal__equal__gt_B) -> SI_call111/2(SI_Y)
  xxRollAutopilotSpec_66_operator/1 -> SI_call111/1(SI_X)
  xxRollAutopilotSpec_71_operator/1 -> SI_call11/2(SI_Y)
  xxRollAutopilotSpec_75_operator/1 -> SI_call11/1(SI_X)
  xxRollAutopilotSpec_11_operator/1(A_equal__equal__gt_B) -> SI_call1/2(SI_Y)
  xxRollAutopilotSpec_15_operator/1 -> SI_call1/1(SI_X)
  xxRollAutopilotSpec_20_operator/1 -> SI_call/2(SI_Y)
  xxRollAutopilotSpec_24_operator/1 -> SI_call/1(SI_X)
  SI_call111111/1(SI_Z) -> PRE_xxRollAutopilotSpec_93/1
  xxRollAutopilotSpec_88_operator/1 -> PRE_xxRollAutopilotSpec_89/1
  xxRollAutopilotSpec_83_operator/1 -> PRE_xxRollAutopilotSpec_84/1
  xxRollAutopilotSpec_7_operator/1 -> PRE_xxRollAutopilotSpec_8/1
  xxRollAutopilotSpec_72_operator/1 -> PRE_xxRollAutopilotSpec_73/1
  xxRollAutopilotSpec_63_operator/1 -> PRE_xxRollAutopilotSpec_64/1
  xxRollAutopilotSpec_58_operator/1 -> PRE_xxRollAutopilotSpec_59/1
  SI_call1111111/1(SI_Z) -> PRE_xxRollAutopilotSpec_42/1
  xxRollAutopilotSpec_37_operator/1 -> PRE_xxRollAutopilotSpec_38/1
  xxRollAutopilotSpec_32_operator/1 -> PRE_xxRollAutopilotSpec_33/1
  xxRollAutopilotSpec_21_operator/1 -> PRE_xxRollAutopilotSpec_22/1
  Ca_operator/1 -> PRE_xxRollAutopilotSpec_184/1
  SI_call11111111/1(SI_Z) -> PRE_xxRollAutopilotSpec_142/1
  xxRollAutopilotSpec_137_operator/1 -> PRE_xxRollAutopilotSpec_138/1
  xxRollAutopilotSpec_132_operator/1 -> PRE_xxRollAutopilotSpec_133/1
  xxRollAutopilotSpec_12_operator/1 -> PRE_xxRollAutopilotSpec_13/1
  xxRollAutopilotSpec_122_operator/1 -> PRE_xxRollAutopilotSpec_123/1
  xxRollAutopilotSpec_113_operator/1 -> PRE_xxRollAutopilotSpec_114/1
  xxRollAutopilotSpec_108_operator/1 -> PRE_xxRollAutopilotSpec_109/1
  xxRollAutopilotSpec_148_operator/1(A_equal__equal__gt_B) -> H_call11/1(H_X)
  xxRollAutopilotSpec_99_operator/1(A_equal__equal__gt_B) -> H_call1/1(H_X)
  xxRollAutopilotSpec_48_operator/1(A_equal__equal__gt_B) -> H_call/1(H_X)
  xxRollAutopilotSpec_177_operator/1 -> Cd_operator/2
  xxRollAutopilotSpec_180_operator/1 -> Cd_operator/1
  Cc_rhs_2/1 -> Cc_operator/2
  xxRollAutopilotSpec_173_operator/1 -> Cb_operator/2
  xxRollAutopilotSpec_174_operator/1 -> Cb_operator/1
  xxRollAutopilotSpec_182_operator/1 -> Ca_operator/1
  xxRollAutopilotSpec_183_ni_3_init/1 -> Arrow_xxRollAutopilotSpec_183_ni_3/1
  xxRollAutopilotSpec_165_ni_16_init/1 -> Arrow_xxRollAutopilotSpec_165_ni_16/1
  xxRollAutopilotSpec_164_ni_12_init/1 -> Arrow_xxRollAutopilotSpec_164_ni_12/1
  xxRollAutopilotSpec_163_ni_9_init/1 -> Arrow_xxRollAutopilotSpec_163_ni_9/1
  xxRollAutopilotSpec_162_ni_7_init/1 -> Arrow_xxRollAutopilotSpec_162_ni_7/1
  spec621_operator/1 -> AP_minus_007/1(In1)
  spec252_operator/1(A_equal__equal__gt_B) -> AP_minus_003D/1(In1)
  branch_14_IF/1 -> AP_minus_003C/1(In1)
  branch_12_IF/1 -> AP_minus_003B/1(In1)
  branch_11_IF/1 -> AP_minus_003A/1(In1)
  spec206_operator/1(A_equal__equal__gt_B) -> AP_minus_001/1(In1)
  RollAutopilotSpec_HDGmode/1 -> no_other_lateral_mode_operator/1, hdg_hold_mode_require_cond/1
  roll_hold_operator/1 -> xxRollAutopilotSpec_15_operator/1, xxRollAutopilotSpec_10_operator/1, xxRollAutopilotSpec_18_operator/1, xxRollAutopilotSpec_24_operator/1, xxRollAutopilotSpec_45_operator/1, xxRollAutopilotSpec_66_operator/1, xxRollAutopilotSpec_61_operator/1, xxRollAutopilotSpec_69_operator/1, xxRollAutopilotSpec_75_operator/1, xxRollAutopilotSpec_96_operator/1, xxRollAutopilotSpec_116_operator/1, xxRollAutopilotSpec_111_operator/1, xxRollAutopilotSpec_119_operator/1, xxRollAutopilotSpec_125_operator/1, xxRollAutopilotSpec_145_operator/1, xxRollAutopilotSpec_91_operator/1, xxRollAutopilotSpec_86_operator/1, PRE_xxRollAutopilotSpec_144/1, PRE_xxRollAutopilotSpec_118/1, PRE_xxRollAutopilotSpec_17/1, PRE_xxRollAutopilotSpec_44/1, PRE_xxRollAutopilotSpec_68/1, xxRollAutopilotSpec_113_operator/1, xxRollAutopilotSpec_108_operator/1, xxRollAutopilotSpec_122_operator/1, xxRollAutopilotSpec_12_operator/1, xxRollAutopilotSpec_132_operator/1, xxRollAutopilotSpec_137_operator/1, xxRollAutopilotSpec_135_operator/1, xxRollAutopilotSpec_140_operator/1, xxRollAutopilotSpec_21_operator/1, xxRollAutopilotSpec_32_operator/1, xxRollAutopilotSpec_37_operator/1, xxRollAutopilotSpec_35_operator/1, xxRollAutopilotSpec_40_operator/1, xxRollAutopilotSpec_58_operator/1, xxRollAutopilotSpec_63_operator/1, xxRollAutopilotSpec_72_operator/1, xxRollAutopilotSpec_7_operator/1, xxRollAutopilotSpec_83_operator/1, xxRollAutopilotSpec_88_operator/1, PRE_xxRollAutopilotSpec_95/1
  Cd_operator/1 -> xxRollAutopilotSpec_29_operator/2, xxRollAutopilotSpec_182_operator/2, xxRollAutopilotSpec_4_operator/2
  Cc_operator/1 -> xxRollAutopilotSpec_28_operator/2, xxRollAutopilotSpec_181_operator/2, xxRollAutopilotSpec_3_operator/2
  Cb_operator/1 -> xxRollAutopilotSpec_28_operator/1, xxRollAutopilotSpec_181_operator/1, xxRollAutopilotSpec_3_operator/1
  Arrow_xxRollAutopilotSpec_183_ni_3/1 -> branch_16_IF/2, branch_15_IF/2
  RollAutopilotSpec_roll_hold_reference/1 -> xxRollAutopilotSpec_152_operator/1, spec216_operator/2, xxRollAutopilotSpec_27_operator/1, xxRollAutopilotSpec_129_operator/1, xxRollAutopilotSpec_78_operator/1, xxRollAutopilotSpec_105_operator/1, xxRollAutopilotSpec_53_operator/1, xxRollAutopilotSpec_2_operator/1
  RollAutopilotSpec_roll_cmd/1 -> spec223_operator/1, spec216_operator/1
  RollAutopilotSpec_TurnKnob/1 -> xxRollAutopilotSpec_176_operator/1, xxRollAutopilotSpec_175_operator/1, xxRollAutopilotSpec_178_operator/1, xxRollAutopilotSpec_179_operator/1, xxRollAutopilotSpec_153_operator/1, xxRollAutopilotSpec_152_operator/2, xxRollAutopilotSpec_154_operator/1, xxRollAutopilotSpec_156_operator/1, xxRollAutopilotSpec_157_operator/1
  branch_13_IF/1 -> xxRollAutopilotSpec_128_operator/2, xxRollAutopilotSpec_104_operator/2
  branch_10_IF/1 -> xxRollAutopilotSpec_23_operator/1, xxRollAutopilotSpec_14_operator/1, xxRollAutopilotSpec_43_operator/1, xxRollAutopilotSpec_9_operator/1, xxRollAutopilotSpec_65_operator/1, xxRollAutopilotSpec_60_operator/1, xxRollAutopilotSpec_74_operator/1, xxRollAutopilotSpec_94_operator/1, xxRollAutopilotSpec_115_operator/1, xxRollAutopilotSpec_110_operator/1, xxRollAutopilotSpec_124_operator/1, xxRollAutopilotSpec_143_operator/1, xxRollAutopilotSpec_90_operator/1, xxRollAutopilotSpec_85_operator/1, xxRollAutopilotSpec_139_operator/1, xxRollAutopilotSpec_134_operator/1, xxRollAutopilotSpec_34_operator/1, xxRollAutopilotSpec_39_operator/1
  xxRollAutopilotSpec_169_operator/1 -> branch_9_IF/2, branch_13_IF/2
  branch_9_IF/1 -> xxRollAutopilotSpec_130_operator/1, xxRollAutopilotSpec_106_operator/1, Cc_operator/1
  RollAutopilotSpec_roll_angle/1 -> xxRollAutopilotSpec_170_operator/1, xxRollAutopilotSpec_169_operator/1, xxRollAutopilotSpec_2_operator/2, xxRollAutopilotSpec_173_operator/1, xxRollAutopilotSpec_174_operator/1, xxRollAutopilotSpec_55_operator/1, xxRollAutopilotSpec_54_operator/1, xxRollAutopilotSpec_80_operator/1, xxRollAutopilotSpec_79_operator/1, xxRollAutopilotSpec_27_operator/2, PRE_xxRollAutopilotSpec_187/1, branch_9_IF/1
  RollAutopilotSpec_autopilot_engaged/1 -> xxRollAutopilotSpec_161_operator/1, spec211_operator/2, roll_hold_operator/2
  no_other_lateral_mode_operator/1 -> spec211_operator/1, roll_hold_operator/1
  RollAutopilotSpec_roll_actuator_command/1 -> xxRollAutopilotSpec_168_operator/1, xxRollAutopilotSpec_167_operator/1, xxRollAutopilotSpec_160_operator/1, branch_8_IF/1
